simulink subsystem "Multisine"  (R2025a)
settings: Solver=VariableStepAuto  StartTime=0.0  StopTime=10.0  RelTol=1e-3
undefined symbols (not defined in the file): MS
settings Model: Creator=17036  LastModifiedBy=gurt1

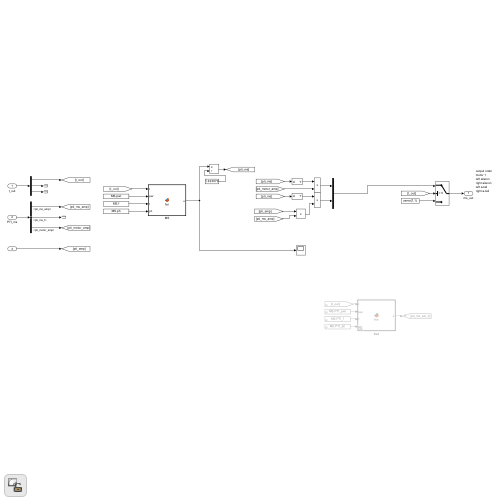
[thumbnail: Simulink's stored preview of the top-level diagram]
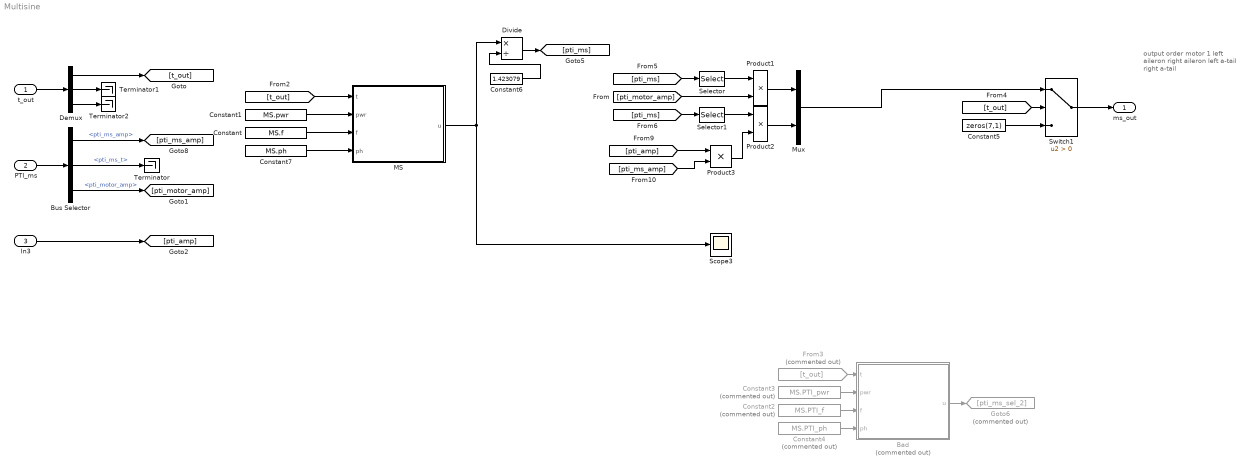
== system Multisine ==
  note: output order
      | motor 1
      | left aileron
      | right aileron
      | left a-tail
      | right a-tail
  t_out : Inport
  PTI_ms : Inport  Port=2
  In3 : Inport  Port=3
  Bad : MATLAB Function  Commented=on  TreatAsAtomicUnit=on
  Bus Selector : BusSelector  OutputSignals=pti_ms_amp,pti_ms_t,pti_motor_amp
  Constant : Constant  Value=MS.f
  Constant1 : Constant  Value=MS.pwr
  Constant2 : Constant  Commented=on  Value=MS.PTI_f
  Constant3 : Constant  Commented=on  Value=MS.PTI_pwr
  Constant4 : Constant  Commented=on  Value=MS.PTI_ph
  Constant5 : Constant  Value=zeros(7,1)
  Constant6 : Constant  Value=1.423079  SampleTime=-1
  Constant7 : Constant  Value=MS.ph
  Demux : Demux  Outputs=3
  Divide : Product  Inputs=*/
  From3 : From  Commented=on  GotoTag=t_out
  Goto6 : Goto  Commented=on  GotoTag=pti_ms_sel_2
  MS : MATLAB Function  TreatAsAtomicUnit=on
  Mux : Mux  Inputs=2
  Product1 : Product
  Product2 : Product
  Product3 : Product
  Scope3 : Scope
      settings: ActiveDisplayYMinimum=-2.51953125  ActiveDisplayYMaximum=1.2109375  DataLoggingVariableName=ScopeData20
  Selector : Selector  InputPortWidth=5  IndexOptions=Index vector (dialog)  Indices=5  OutputSizes=1
  Selector1 : Selector  InputPortWidth=5  IndexOptions=Index vector (dialog)  Indices=[1:4]  OutputSizes=1
  Switch1 : Switch  Criteria=u2 > Threshold  SaturateOnIntegerOverflow=off  InputSameDT=off
  Terminator : Terminator
  Terminator1 : Terminator
  Terminator2 : Terminator
  ms_out : Outport
  wires:
  PTI_ms/1 -> Bus Selector/1
  Bus Selector/1 -> [pti_ms_amp]  "<pti_ms_amp>"
  Switch1/1 -> ms_out/1
  t_out/1 -> Demux/1
  Demux/2 -> Terminator1/1
  Bus Selector/2 -> Terminator/1  "<pti_ms_t>"
  Bad/1(u) -> Goto6/1
  Constant2/1 -> Bad/3(f)
  Constant4/1 -> Bad/4(ph)
  From3/1 -> Bad/1(t)
  Constant3/1 -> Bad/2(pwr)
  [t_out] -> Switch1/2
  Constant5/1 -> Switch1/3
  Demux/1 -> [t_out]
  Demux/3 -> Terminator2/1
  Bus Selector/3 -> [pti_motor_amp]  "<pti_motor_amp>"
  [pti_ms] -> Selector/1
  [pti_motor_amp] -> Product1/2
  Selector/1 -> Product1/1
  [pti_ms] -> Selector1/1
  Product1/1 -> Mux/1
  Selector1/1 -> Product2/1
  Product2/1 -> Mux/2
  In3/1 -> [pti_amp]
  [t_out] -> MS/1(t)
  Constant1/1 -> MS/2(pwr)
  Constant/1 -> MS/3(f)
  Constant7/1 -> MS/4(ph)
  [pti_amp] -> Product3/1
  [pti_ms_amp] -> Product3/2
  Product3/1 -> Product2/2
  MS/1(u) -> Scope3/1, Divide/1
  Mux/1 -> Switch1/1
  Constant6/1 -> Divide/2
  Divide/1 -> [pti_ms]

== matlab function Multisine/Bad ==
  data: t input; u output; pwr input; f input; ph input
function u  = fcn(t,pwr,f,ph)

[nf,ni] = size(f);

u = zeros(ni,1);
t = double(t);

for jj=1:ni
    for kk = 1:nf
        u(jj) = u(jj)+sqrt(pwr(kk,jj))*sin(2*pi*f(kk,jj)*t+ph(kk,jj));
        %sin(2*pi*f(kk,jj)*t)
    end
end

== matlab function Multisine/MS ==
  data: t input; u output; pwr input; f input; ph input
function u  = fcn(t,pwr,f,ph)

[nf,ni] = size(f);

u = zeros(ni,1);
t = double(t);

for jj=1:ni
    for kk = 1:nf
        u(jj) = u(jj)+sqrt(pwr(kk,jj))*sin(2*pi*f(kk,jj)*t+ph(kk,jj));
    end
end
